simulink model "modeleaminesbeh"  (R2023a)
settings: Solver=VariableStepAuto  StartTime=0.0  StopTime=15  RelTol=1e-3
InitFcn:
  | Rm=3.15;
  | Lm=0.0015;
  | K=1.028;
  | fm=0.16805;
  | A2=0.0033153;
  | A1=0.045721;
  | L01=0.2625;
  | m2=0.24355;
  | A1tilde=A1+A2+m2*L01*L01;
  | A2tilde=A1tilde-A2;
  | f=0.070633;
  | lg1=0.16655703376925832;
  | m1=0.66984;
  | g=9.8;
  | Ceq=L01*m2*g+lg1*m1*g;
settings Model: Creator=mimom  LastModifiedBy=mimom

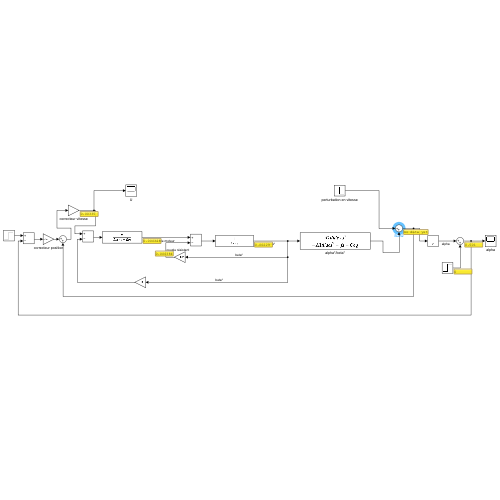
[thumbnail: Simulink's stored preview of the top-level diagram]
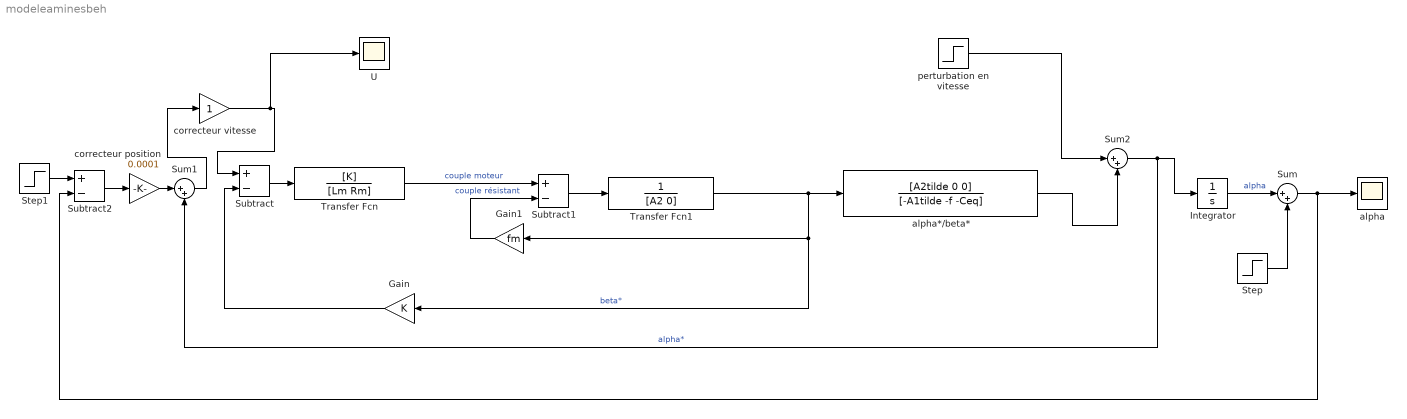
== system modeleaminesbeh ==
  Gain : Gain  Gain=K
  Gain1 : Gain  Gain=fm
  Integrator : Integrator
  Step : Step  Time=0.01  After=0  SampleTime=0
  Step1 : Step  Time=10  After=0  SampleTime=0
  Subtract : Sum  Inputs=+-
  Subtract1 : Sum  Inputs=+-
  Subtract2 : Sum  Inputs=+-
  Sum : Sum  Inputs=|++
  Sum1 : Sum  Inputs=|++
  Sum2 : Sum  Inputs=|++
  Transfer Fcn : TransferFcn  Numerator=[K]  Denominator=[Lm Rm]
  Transfer Fcn1 : TransferFcn  Denominator=[A2 0]
  U : Scope
  alpha : Scope
  alpha*/beta* : TransferFcn  Numerator=[A2tilde 0 0]  Denominator=[-A1tilde -f -Ceq]
  correcteur position : Gain  Gain=0.0001
  correcteur vitesse : Gain
  perturbation en vitesse : Step  Time=0.5  Before=1  After=0  SampleTime=0
  wires:
  Gain/1 -> Subtract/2
  Subtract/1 -> Transfer Fcn/1
  Transfer Fcn/1 -> Subtract1/1  "couple moteur"
  Subtract1/1 -> Transfer Fcn1/1
  Transfer Fcn1/1 -> alpha*/beta*/1, Gain/1, Gain1/1  "beta*"
  Step/1 -> Sum/2
  Step1/1 -> Subtract2/1
  Subtract2/1 -> correcteur position/1
  Sum/1 -> Subtract2/2, alpha/1
  Gain1/1 -> Subtract1/2  "couple résistant"
  Sum1/1 -> correcteur vitesse/1
  correcteur vitesse/1 -> U/1, Subtract/1
  correcteur position/1 -> Sum1/1
  Integrator/1 -> Sum/1  "alpha"
  Sum2/1 -> Sum1/2, Integrator/1  "alpha*"
  alpha*/beta*/1 -> Sum2/2
  perturbation en vitesse/1 -> Sum2/1
